simulink model "Prob_2_model"  (R2016a)
settings: Solver=VariableStepAuto  StartTime=0.0  StopTime=100  RelTol=1e-3
values from neighbouring files (symbols this model uses):
  b = 50    [MAT_file.mat]
  k1 = 50    [MAT_file.mat]
  k2 = 250    [MAT_file.mat]
  M1 = 800    [MAT_file.mat]
  M2 = 25    [MAT_file.mat]
settings Model: Creator=Admin  LastModifiedBy=Admin

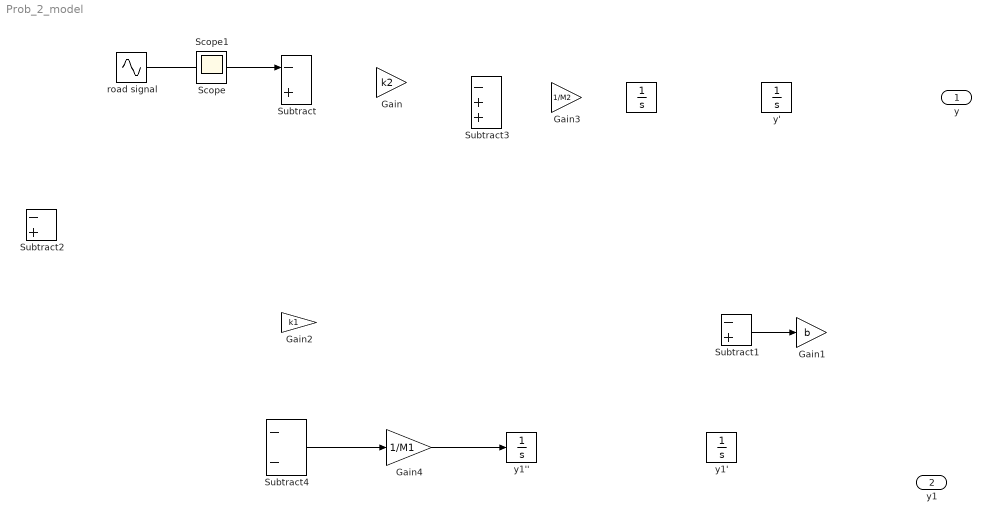
== system Prob_2_model ==
  " " : Integrator
  Gain : Gain  Gain=k2
  Gain1 : Gain  Gain=b
  Gain2 : Gain  Gain=k1
  Gain3 : Gain  Gain=1/M2
  Gain4 : Gain  Gain=1/M1
  Subtract : Sum  Inputs=-+
  Subtract1 : Sum  Inputs=-+
  Subtract2 : Sum  Inputs=-+
  Subtract3 : Sum  Inputs=-++
  Subtract4 : Sum  Inputs=--
  road signal : Sin  SampleTime=0
  y' : Integrator
  y1' : Integrator
  y1'' : Integrator
  "y " : Outport
  "y1 " : Outport  Port=2
  Scope : Scope
  Scope1 : Scope
  wires:
  Subtract1/1 -> Gain1/1
  Gain4/1 -> y1''/1
  Subtract4/1 -> Gain4/1
  road signal/1 -> Subtract/1
